simulink model "practice10_1"  (Simulink 7.9)
settings: Solver=ode45  StartTime=0.0  StopTime=10.0  RelTol=1e-3
settings Model: Creator=sony  LastModifiedBy=sony

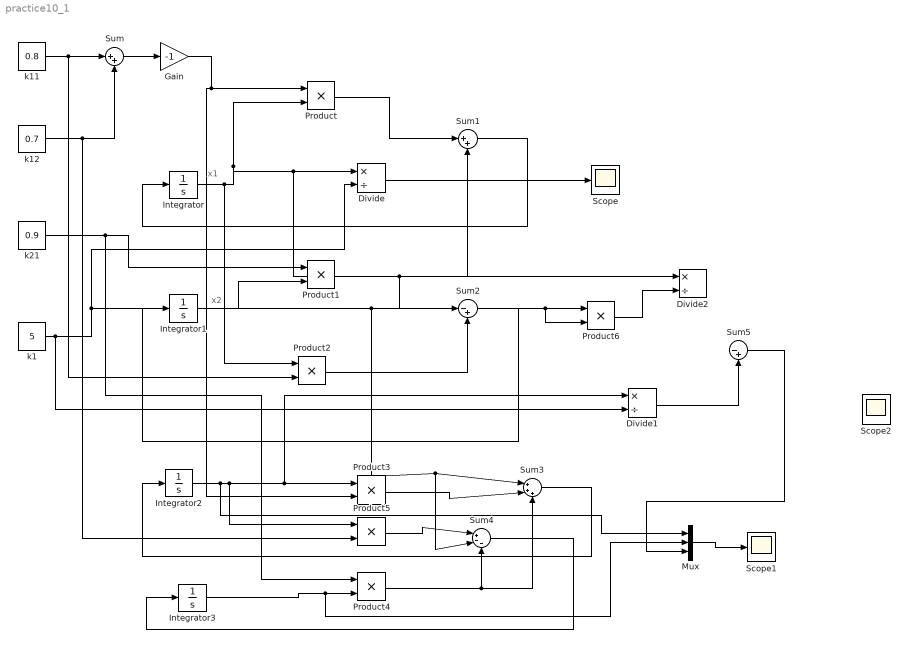
== system practice10_1 ==
  note: x1
  note: x2
  Divide : Product  Inputs=*/
  Divide1 : Product  Inputs=*/
  Divide2 : Product  Inputs=*/
  Gain : Gain  Gain=-1
  Integrator : Integrator  InitialCondition=200
  Integrator1 : Integrator
  Integrator2 : Integrator
  Integrator3 : Integrator
  Mux : Mux  Inputs=3
  Product{,1..6} (7 alike) : Product  RndMeth=Zero
  Scope : Scope
  Scope1 : Scope
  Scope2 : Scope
      settings: SaveName=ScopeData2
  Sum : Sum  Inputs=|++
  Sum1 : Sum  Inputs=|++
  Sum2 : Sum  Inputs=|-+
  Sum3 : Sum  Inputs=|+++
  Sum4 : Sum  Inputs=|+--
  Sum5 : Sum  Inputs=|-+
  k1 : Constant  Value=5
  k11 : Constant  Value=0.8
  k12 : Constant  Value=0.7
  k21 : Constant  Value=0.9
  wires:
  k11/1 -> Sum/1, Product2/2
  k12/1 -> Sum/2, Product5/2
  Sum/1 -> Gain/1
  Integrator/1 -> Product2/1, Product/2, Divide/1, Divide2/1
  k21/1 -> Product1/1, Product4/1
  Integrator1/1 -> Product1/2
  Product/1 -> Sum1/1
  Product1/1 -> Sum1/2, Sum2/1
  Sum1/1 -> Integrator/1
  Product2/1 -> Sum2/2
  Sum2/1 -> Integrator1/1
  k1/1 -> Divide1/2, Divide/2, Product6/1, Product6/2, Sum3/1, Sum4/2
  Divide/1 -> Scope/1
  Gain/1 -> Product/1, Product3/2
  Integrator2/1 -> Product5/1, Product3/1, Divide1/1, Mux/1
  Product3/1 -> Sum3/2
  Sum3/1 -> Integrator2/1
  Product5/1 -> Sum4/1
  Mux/1 -> Scope1/1
  Integrator3/1 -> Product4/2, Mux/2
  Product4/1 -> Sum3/3, Sum4/3
  Sum4/1 -> Integrator3/1
  Divide1/1 -> Sum5/2
  Product6/1 -> Divide2/2
  Sum5/1 -> Mux/3
